simulink subsystem "Elasped_Time"  (R2024b)
settings: Solver=VariableStepAuto  StartTime=0.0  StopTime=10.0  RelTol=1e-3
undefined symbols (not defined in the file): FCS
libraries: simulink x2
settings Model: Creator=bmsimmon  LastModifiedBy=macheson
settings RTWCC: GPUComputeCapability=3.5

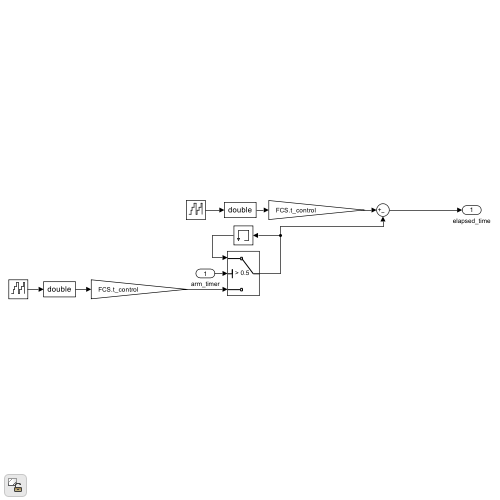
[thumbnail: Simulink's stored preview of the top-level diagram]
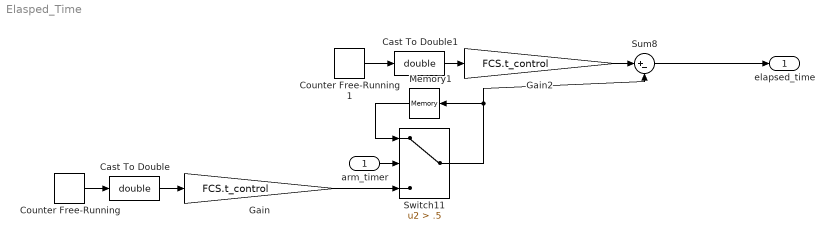
== system Elasped_Time ==
  arm_timer : Inport
  Cast To Double : DataTypeConversion  OutDataTypeStr=double  SaturateOnIntegerOverflow=off  RndMeth=Floor
  Cast To Double1 : DataTypeConversion  OutDataTypeStr=double  SaturateOnIntegerOverflow=off  RndMeth=Floor
  Counter Free-Running : simulink/Sources/Counter Free-Running  NumBits=32  tsamp=-1
  Counter Free-Running1 : simulink/Sources/Counter Free-Running  NumBits=32  tsamp=-1
  Gain : Gain  Gain=FCS.t_control  OutDataTypeStr=double
  Gain2 : Gain  Gain=FCS.t_control  OutDataTypeStr=double
  Memory1 : Memory
  Sum8 : Sum  Inputs=|+-
  Switch11 : Switch  Criteria=u2 > Threshold  Threshold=.5  SaturateOnIntegerOverflow=off  InputSameDT=off
  elapsed_time : Outport
  wires:
  Cast To Double/1 -> Gain/1
  Memory1/1 -> Switch11/1
  arm_timer/1 -> Switch11/2
  Gain2/1 -> Sum8/1
  Switch11/1 -> Memory1/1, Sum8/2
  Gain/1 -> Switch11/3
  Counter Free-Running/1 -> Cast To Double/1
  Counter Free-Running1/1 -> Cast To Double1/1
  Sum8/1 -> elapsed_time/1
  Cast To Double1/1 -> Gain2/1
